simulink model "atrias_nmm_hardware"  (R2014b)
settings: Solver=FixedStepDiscrete  StartTime=0.0  StopTime=inf  FixedStep=sample_time  RelTol=1e-3
undefined symbols (not defined in the file or in its folder): A_lpf_dtau, B1_lpf_dtau, B2_lpf_dtau, boom_mount_angle, boom_pelvis_offset_angle, c, c_jointstop, contactThr, control_start_time, D12_T, d_y_boom_com_offset, d_y_boom_hip_offset, eref, fcut_contact, FmaxBFSH, FmaxGLU, FmaxHAM, FmaxHFL, FmaxRF, FmaxVAS, g, h_boom, HIP_MTR_MAX_CONT_TORQUE, initial_com_height, initial_dx, K, k_sea, kd_lateral, kp_lateral, l_boom_projected, L_distribution_switch, L_hip_trq_desired, L_knee_trq_desired, L_sea_ctrl_switch, l_seg, L_stim_gain, L_stim_switch, l_yaw_center_to_pelvis, lambdaHip, lambdaKnee, lateral_offset, lateral_target_angle_left, lateral_target_angle_right, lateral_transition_force, loptBFSH, loptGLU, loptHAM, loptHFL, loptRF, loptVAS, lslackBFSH, lslackGLU, lslackHAM, lslackHFL, lslackRF, lslackVAS, LStim_Constant, m_leg_motor, m_total_real, max_torque_lateral ... (+59)
libraries: simulink x5, simulink_extras x3, slrtlib x3
(part 1 of 4)
settings Model: BufferReuse=off  Creator=wmartin  LastModifiedBy=ryan
settings SolverCC: EnableConcurrentExecution=on
settings DataIOCC: MaxDataPoints=1000000000  SaveFormat=StructureWithTime
settings OptimizationCC: BlockReduction=off  OptimizeBlockIOStorage=off  BufferReuse=off  GlobalBufferReuse=off  ExpressionFolding=off  ExpressionDepthLimit=2147483647  LocalBlockOutputs=off  SimCompilerOptimization=On
settings DebuggingCC: UnderspecifiedInitializationDetection=Classic  MergeDetectMultiDrivingBlocksExec=none  StateNameClashWarn=warning
settings HardwareCC: ProdIntDivRoundTo=Zero  ProdEndianess=LittleEndian  ProdLongLongMode=on  ProdHWDeviceType=Generic->32-bit x86 compatible
settings ModelReferenceCC: UpdateModelReferenceTargets=IfOutOfDate  EnableParallelModelReferenceBuilds=on
settings RTWCC: SystemTargetFile=slrt.tlc  TemplateMakefile=slrt_default_tmf  Description=Simulink Real-Time  RTWVerbose=off  ProcessScript=slrt_make_rtw_hook  RTWCompilerOptimization=On
settings CodeAppCC: MaxIdLength=256
settings SimulinkRealTimeCC: GeneratePreprocessorConditionals=Disable all  EnableShiftOperators=on  RL32LogBufSizeModifier=100000000

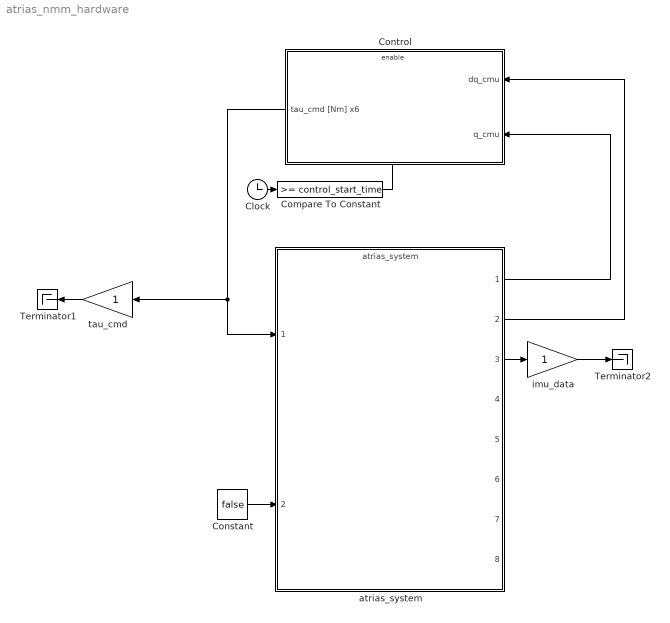
== system atrias_nmm_hardware ==
  Clock : Clock
  Compare To Constant : simulink/Logic and Bit Operations/Compare To Constant  relop=>=  const=control_start_time  OutDataTypeStr=boolean
  Constant : Constant  Value=false
  Control : Subsystem
  Terminator1 : Terminator
  Terminator2 : Terminator
  atrias_system : ModelReference  ModelNameDialog=atrias_system  SimulationMode=Normal  ModelReferenceVersion=1.2605  CopyOfModelName=atrias_system  DefaultDataLogging=on
  imu_data : Gain
  tau_cmd : Gain
  wires:
  Clock/1 -> Compare To Constant/1
  Compare To Constant/1 -> Control/Enable
  atrias_system/1 -> Control/2(q_cmu)
  atrias_system/2 -> Control/1(dq_cmu)
  Constant/1 -> atrias_system/2
  Control/1(tau_cmd [Nm] x6) -> tau_cmd/1, atrias_system/1
  imu_data/1 -> Terminator2/1
  atrias_system/3 -> imu_data/1
  tau_cmd/1 -> Terminator1/1

== system atrias_nmm_hardware/Control ==
  dq_cmu : Inport
  q_cmu : Inport  Port=2
  Enable : EnablePort  StatesWhenEnabling=reset
  Actuator Control : ModelReference  ModelNameDialog=actuator_control  SimulationMode=Normal  ModelReferenceVersion=1.66  CopyOfModelName=actuator_control  DefaultDataLogging=on
  Behavior Control : Subsystem
  tau_cmd [Nm] x6 : Outport  InitialOutput=[0 0 0 0 0 0]
  wires:
  q_cmu/1 -> Actuator Control/4, Behavior Control/2(q_cmu)
  dq_cmu/1 -> Actuator Control/5, Behavior Control/1(dq_cmu)
  Behavior Control/1(Motor Torque Command [Nm] x6) -> Actuator Control/1
  Actuator Control/1 -> tau_cmd [Nm] x6/1
  Behavior Control/2(SEA Torque Velocity Command [Nm] x4) -> Actuator Control/2
  Behavior Control/3(Force / Position Control [1/0] x4) -> Actuator Control/3

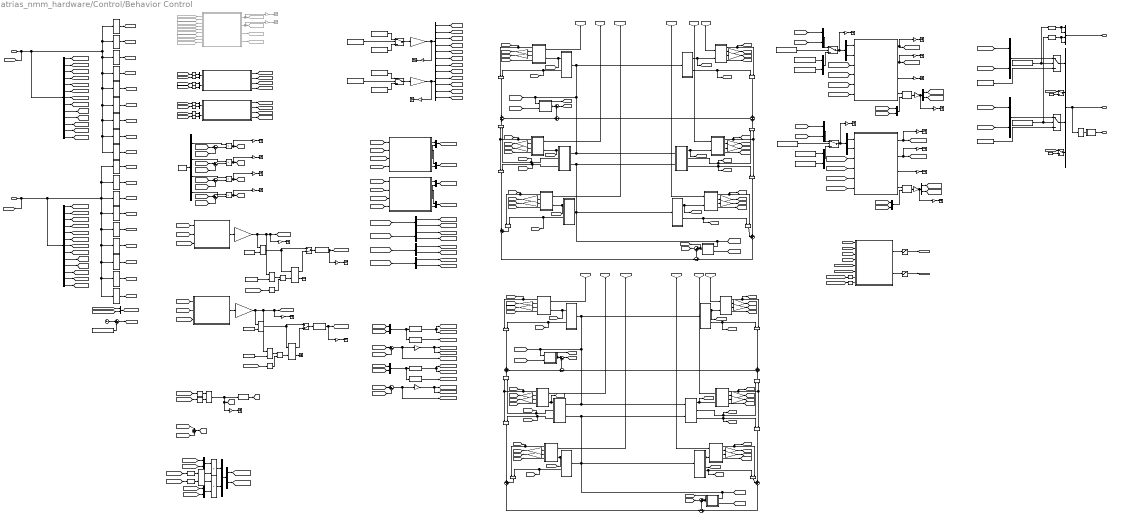
== system atrias_nmm_hardware/Control/Behavior Control ==
  note: Velocity Estimation
  note: Muscle Stimulation Input
  note: Leg/Spring Measurements
  note: Lateral Behavior
  note: Torque Commands
  note: Inputs
  note: q Order:
      |
      | backJointR
      | backGearR
      | frontJointR
      | frontGearR
      |
      | backJointL
      | backGearL
      | frontJointL
      | frontGearL
      |
      | latR
      | latL
      |
      | boomRoll
      | boomYaw
      | boomPitch
  note: Motor Order:
      |
      | backR
      | frontR
      | latR
      | backL
      | frontL
      | latL
  note: Muscle Geometry Input
  note: Atrias Knee/Splay Angles
  note: Estimate SEA Torque
  note: Estimate Leg Load and Contact
  note: Hip/Knee Torque Distribution
  note: Left Leg
  note: Neural Control Layer Interface
  note: Muscle Actuation Layer
  note: Body Mechanics Layer
      | Interface (Left Hip Joint)
  note: Body Mechanics Layer
      | Interface (Left Knee Joint)
  note: Right Leg
  note: Neural Control Layer Interface
  note: Body Mechanics Layer
      | Interface (Left Hip Joint)
  note: Body Mechanics Layer
      | Interface (Left Knee Joint)
  note: Estimate Flight/Escape
  note: Estimate GRFy
  note: Estimate Primary Leg Length/Angle
  dq_cmu : Inport
  q_cmu : Inport  Port=2
  Clock : Clock
  Constant : Constant  Value=0
  Constant1 : Constant  Value=0
  Constant10 : Constant  Value=releaseThr
  Constant11 : Constant  Value=contactThr
  Constant12 : Constant  Value=releaseThr
  Constant13 : Constant  Value=L_knee_trq_desired
  Constant14 : Constant  Value=R_knee_trq_desired
  Constant15 : Constant  Value=R_distribution_switch
  Constant16 : Constant  Value=L_distribution_switch
  Constant17 : Constant  Value=R_sea_ctrl_switch
  Constant18 : Constant  Value=L_sea_ctrl_switch
  Constant19 : Constant  Value=[0;0]
  Constant2 : Constant  Value=control_start_time
  Constant20 : Constant  Value=[0;0]
  Constant21 : Constant  Value=R_hip_trq_desired
  Constant22 : Constant  Value=L_hip_trq_desired
  Constant23 : Constant  Value=k_sea
  Constant3 : Constant  Value=LStim_Constant
  Constant4 : Constant  Value=RStim_Constant
  Constant5 : Constant  Value=[0;0;0;0;0;0]
  Constant6 : Constant  Value=[0;0;0;0;0;0]
  Constant7 : Constant  Value=R_stim_switch
  Constant8 : Constant  Value=L_stim_switch
  Constant9 : Constant  Value=contactThr
  Data Type Conversion : DataTypeConversion  OutDataTypeStr=double
  Data Type Conversion1 : DataTypeConversion  OutDataTypeStr=double
  Data Type Conversion{2..5} (4 alike) : DataTypeConversion  OutDataTypeStr=boolean
  Demux{,1,3,14..19} (9 alike) : Demux  Outputs=2
  Demux11 : Demux  Outputs=6
  Demux12 : Demux  Outputs=13
  Demux13 : Demux  Outputs=13
  Demux2 : Demux  Outputs=6
  Demux4 : Demux
  Detect Increase : simulink/Logic and Bit Operations/Detect Increase  vinit=0.0  InputProcessing=Inherited  OutDataTypeStr=boolean
  From116 : From  Commented=on  GotoTag=qBoomYaw
  From22 : From  Commented=on  GotoTag=GRFy
  From28 : From  Commented=on  GotoTag=dqBoomYaw
  From29 : From  Commented=on  GotoTag=qBoomRoll
  From45 : From  Commented=on  GotoTag=TorsoPitch
  From50 : From  Commented=on  GotoTag=PrimaryLegAngle
  From51 : From  Commented=on  GotoTag=PrimaryLegLength
  From52 : From  Commented=on  GotoTag=dqBoomRoll
  From81 : From  Commented=on  GotoTag=escape
  GLU Link : Subsystem
  GLU Link1 : Subsystem
  Gain : Gain
  Gain1 : Gain  Gain=R_stim_gain
  Gain2 : Gain  Gain=-1
  Gain3 : Gain  Gain=L_stim_gain
  Gain4 : Gain
  Gain5 : Gain  Gain=-1
  Goto26 : Goto  Commented=on  GotoTag=dx_avg
  Goto48 : Goto  Commented=on  GotoTag=dy_avg
  Goto49 : Goto  Commented=on  GotoTag=tApex
  Goto50 : Goto  Commented=on  GotoTag=systemEnergy
  HAM Link : Subsystem
  HAM Link1 : Subsystem
  HFL Link : Subsystem
  HFL Link1 : Subsystem
  L BFSH : Subsystem
  L BFSH Link : Subsystem
  L BFSH Link1 : Subsystem
  L GLU : Subsystem
  L Geometry : Subsystem
  L HAM : Subsystem
  L HFL : Subsystem
  L HFL Muscle Spindles{,1,4..5} (4 alike) : Gain  Gain=1/loptHFL
  L HFL Muscle Spindles{2..3,6..7} (4 alike) : Gain  Gain=1/loptGLU
  L Hip Joint Limits : Subsystem
  L Hip Joint Limits1 : Subsystem
  L Knee Joint Limits : Subsystem
  L Knee Joint Limits1 : Subsystem
  L Leg Calculator : Subsystem
  L Leg Load : Subsystem
  L RF : Subsystem
  L RF Muscle Spindles{,1..3} (4 alike) : Gain  Gain=1/loptRF
  L RF Muscle Spindles{4..7} (4 alike) : Gain  Gain=1/loptVAS
  L Torque : Subsystem
  L VAS : Subsystem
  LLoad : Gain
  L_Contact : Gain
  L_distribution_constraint_flag : Gain
  L_sea_B_des : Gain
  L_sea_B_meas : Gain
  L_sea_F_des : Gain
  L_sea_F_meas : Gain
  L_stim : Gain
  L_tau_virt_des : Gain
  L_tau_virt_meas : Gain
  Lateral Control : MATLAB Function  TreatAsAtomicUnit=on
  Left Lateral Torque Saturation : Saturate  UpperLimit=max_torque_lateral  LowerLimit=-max_torque_lateral
      settings: AttributesFormatString=Top: %<UpperLimit>\nBottom: %<LowerLimit>
  Logical Operator : Logic  Operator=NOT  AllPortsSameDT=off  OutDataTypeStr=boolean
  Logical Operator1 : Logic  AllPortsSameDT=off  OutDataTypeStr=boolean
  Logical Operator2 : Logic  AllPortsSameDT=off  OutDataTypeStr=boolean
  Logical Operator3 : Logic  Operator=NOT  AllPortsSameDT=off  OutDataTypeStr=boolean
  Logical Operator4 : Logic  AllPortsSameDT=off  OutDataTypeStr=boolean
  Manual Switch : ManualSwitch
  Manual Switch1 : ManualSwitch
  Manual Switch2 : ManualSwitch  CurrentSetting=0
  Manual Switch3 : ManualSwitch  CurrentSetting=0
  Matrix Multiply : Product  Multiplication=Matrix(*)
  Matrix Multiply1 : Product  Multiplication=Matrix(*)
  Memory : Memory
  Memory1 : Memory
  Mux : Mux
  Mux{1..2,4..13,17..18,20..27} (22 alike) : Mux  Inputs=2
  Mux3 : Mux
  Product{,1..3,10..11} (6 alike) : Product
  Product{4..9,12,14..15,17..23} (16 alike) : Product  RndMeth=Zero
  R BFSH : Subsystem
  R GLU : Subsystem
  R Geometry : Subsystem
  R HAM : Subsystem
  R HAM Muscle Spindles{1,3,6,14} (4 alike) : Gain  Gain=1/loptHAM
  R HAM Muscle Spindles{2,4,12..13} (4 alike) : Gain  Gain=1/loptBFSH
  R HFL : Subsystem
  R Leg Calculator : Subsystem
  R Leg Load : Subsystem
  R RF : Subsystem
  R Torque : Subsystem
  R VAS : Subsystem
  RF Link : Subsystem
  RF Link1 : Subsystem
  RLoad : Gain
  R_Contact : Gain
  R_distribution_constraint_flag : Gain
  R_sea_B_des : Gain
  R_sea_B_meas : Gain
  R_sea_F_des : Gain
  R_sea_F_meas : Gain
  R_stim : Gain
  R_tau_virt_des : Gain
  R_tau_virt_meas : Gain
  Relational Operator : RelationalOperator  OutDataTypeStr=boolean
  Relational Operator1 : RelationalOperator  Operator=<=  OutDataTypeStr=boolean
  Relational Operator2 : RelationalOperator  OutDataTypeStr=boolean
  Relational Operator3 : RelationalOperator  Operator=<=  OutDataTypeStr=boolean
  Right Lateral Torque Saturation : Saturate  UpperLimit=max_torque_lateral  LowerLimit=-max_torque_lateral
      settings: AttributesFormatString=Top: %<UpperLimit>\nBottom: %<LowerLimit>
  S-R Flip-Flop : simulink_extras/Flip Flops/S-R Flip-Flop  initial_condition=0
  S-R Flip-Flop1 : simulink_extras/Flip Flops/S-R Flip-Flop  initial_condition=0
  S-R Flip-Flop2 : simulink_extras/Flip Flops/S-R Flip-Flop  initial_condition=0
  Selector{,3,14..17,24..27} (10 alike) : Selector  InputPortWidth=2  Indices=[1]
  Selector1 : Selector  InputPortWidth=13  Indices=[10]
  Selector10 : Selector  InputPortWidth=13  Indices=[7 8]
  Selector11 : Selector  InputPortWidth=13  Indices=[9]
  Selector12 : Selector  InputPortWidth=13  Indices=[1 2]
  Selector13 : Selector  InputPortWidth=13  Indices=[3 4]
  Selector18 : Selector  InputPortWidth=13  Indices=[13]
  Selector2 : Selector  InputPortWidth=13  Indices=[5 6]
  Selector20 : Selector  InputPortWidth=13  Indices=[13]
  Selector21 : Selector  InputPortWidth=13  Indices=[11]
  Selector22 : Selector  InputPortWidth=13  Indices=[12]
  Selector23 : Selector  InputPortWidth=13  Indices=[11]
  Selector28 : Selector  InputPortWidth=13  Indices=[12]
  Selector33 : Selector  InputPortWidth=6  Indices=[1 2 4 5]
  Selector4 : Selector  InputPortWidth=13  Indices=[7 8]
  Selector5 : Selector  InputPortWidth=13  Indices=[9]
  Selector6 : Selector  InputPortWidth=13  Indices=[1 2]
  Selector7 : Selector  InputPortWidth=13  Indices=[3 4]
  Selector8 : Selector  InputPortWidth=13  Indices=[10]
  Selector9 : Selector  InputPortWidth=13  Indices=[5 6]
  Sum{,2,4,6,9,15,20} (7 alike) : Sum  Inputs=|+-
  Sum{1,7,12,16,18,22} (6 alike) : Sum  Inputs=|++
  Sum10 : Sum  Inputs=+-
  Sum{3,8,11,19,23} (5 alike) : Sum
  Sum13 : Sum  Inputs=++|
  Sum14 : Sum  Inputs=+-
  Sum17 : Sum  Inputs=++|
  Sum21 : Sum  Inputs=-+
  Sum5 : Sum  Inputs=-+
  Switch : Switch  Criteria=u2 ~= 0
  Switch1 : Switch  Criteria=u2 ~= 0
  Switch{2..5} (4 alike) : Switch  Criteria=u2 > Threshold
  Terminator : Terminator  Commented=on
  Terminator{1..4,6..24} (23 alike) : Terminator
  Terminator5 : Terminator  Commented=on
  VAS Link : Subsystem
  VAS Link1 : Subsystem
  Velocity Estimation : Subsystem  Commented=on
  "[N] to [%bw]" : Gain  Gain=1/(m_total_real*g)
  dtau_des : Subsystem
  dx_avg : Gain  Commented=on
  dy_avg : Gain  Commented=on
  flight : Gain
  knee angle : Fcn  Expr=pi-(u(1)-u(2))
  knee angle1 : Fcn  Expr=pi-(u(1)-u(2))
  percent body weight : Gain  Gain=1/(m_total_real*g)
  splay angle : Fcn  Expr=(u(1)-u(2))
  splay angle1 : Fcn  Expr=(u(1)-u(2))
  Motor Torque Command [Nm] x6 : Outport  OutputWhenDisabled=reset  InitialOutput=[0 0 0 0 0 0]
  SEA Torque Velocity Command [Nm] x4 : Outport  Port=2  OutputWhenDisabled=reset  InitialOutput=[0 0 0 0 0 0]
  Force / Position Control [1/0] x4 : Outport  Port=3  OutputWhenDisabled=reset  InitialOutput=[0 0 0 0 0 0]
  tag scope: GRFy=global, LActBFSH=global, LActGLU=global, LActHAM=global, LActHFL=global, LActRF=global, LActVAS=global, LFmBFSH=global, LFmGLU=global, LFmHAM=global, LFmHFL=global, LFmRF=global, LFmVAS=global, LFootCnt=global, LHipStop=global, LKneeStop=global, LLLoad=global, LLceBFSH=global, LLceGLU=global, LLceHAM=global, LLceHFL=global, LLceRF=global, LLceVAS=global, LLmtuBFSH=global, LLmtuGLU=global, LLmtuHAM=global, LLmtuHFL=global, LLmtuRF=global, LLmtuVAS=global, LM12=global, LM12_achieved=global, LM23=global, LM23_achieved=global, LStimBFSH=global, LStimGLU=global, LStimHAM=global, LStimHFL=global, LStimRF=global, LStimVAS=global, LVceBFSH=global, LVceGLU=global, LVceHAM=global, LVceHFL=global, LVceRF=global, LVceVAS=global, Ldgear_shin=global, Ldgear_thigh=global, Ldphi12=global, Ldphi23=global, Ldphi_Lat=global, Ldphi_back_knee=global, Ldphi_front_knee=global, Ldphi_lower_splay=global, Ldphi_shin=global, Ldphi_thigh=global, Lgear_shin=global, Lgear_thigh=global, Lphi12=global, Lphi12dphi12=global, Lphi23=global, Lphi23dphi23=global, Lphi_Lat=global, Lphi_back_knee=global, Lphi_front_knee=global, Lphi_lower_splay=global, Lphi_shin=global, Lphi_thigh=global, LrBFSH=global, LrGLU=global, LrHAMh=global, LrHAMk=global, LrHFL=global, LrRFh=global, LrRFk=global, LrVAS=global, Lshin_ctrl_trq=global, LtauB=global, LtauF=global, Lthigh_ctrl_trq=global, RActBFSH=global, RActGLU=global, RActHAM=global, RActHFL=global, RActRF=global, RActVAS=global, RFmBFSH=global, RFmGLU=global, RFmHAM=global, RFmHFL=global, RFmRF=global, RFmVAS=global, RFootCnt=global, RHipStop=global, RKneeStop=global, RLLoad=global, RLceBFSH=global, RLceGLU=global, RLceHAM=global, RLceHFL=global, RLceRF=global, RLceVAS=global, RLmtuBFSH=global, RLmtuGLU=global, RLmtuHAM=global, RLmtuHFL=global, RLmtuRF=global, RLmtuVAS=global, RM12=global, RM12_achieved=global, RM23=global, RM23_achieved=global, RStimBFSH=global, RStimGLU=global, RStimHAM=global, RStimHFL=global, RStimRF=global, RStimVAS=global, RVceBFSH=global, RVceGLU=global, RVceHAM=global, RVceHFL=global, RVceRF=global, RVceVAS=global, Rdgear_shin=global, Rdgear_thigh=global, Rdphi12=global, Rdphi23=global, Rdphi_Lat=global, Rdphi_back_knee=global, Rdphi_front_knee=global, Rdphi_lower_splay=global, Rdphi_shin=global, Rdphi_thigh=global, Rgear_shin=global, Rgear_thigh=global, Rphi12=global, Rphi12dphi12=global, Rphi23=global, Rphi23dphi23=global, Rphi_Lat=global, Rphi_back_knee=global, Rphi_front_knee=global, Rphi_lower_splay=global, Rphi_shin=global, Rphi_thigh=global, RrBFSH=global, RrGLU=global, RrHAMh=global, RrHAMk=global, RrHFL=global, RrRFh=global, RrRFk=global, RrVAS=global, Rshin_ctrl_trq=global, RtauB=global, RtauF=global, Rthigh_ctrl_trq=global, droll=global, dtheta=global, dyaw=global, escape=global, flight=global, roll=global, theta=global, yaw=global
  wires:
  Switch1/1 -> Mux/3
  Mux18/1 -> Switch1/1
  Constant19/1 -> Switch/3
  Mux17/1 -> Switch/1
  [Lthigh_ctrl_trq] -> Mux18/2
  [Lshin_ctrl_trq] -> Mux18/1
  [Rshin_ctrl_trq] -> Mux17/1
  [Rthigh_ctrl_trq] -> Mux17/2
  Manual Switch/1 -> Mux/4
  Manual Switch1/1 -> Mux/2
  Switch/1 -> Mux/1
  Constant18/1 -> Switch1/2, Data Type Conversion3/1
  Constant17/1 -> Switch/2, Data Type Conversion2/1
  Mux3/1 -> Force / Position Control [1/0] x4/1
  Mux7/1 -> [TorsoPitch]
  [dqBoomPitch] -> Mux7/2
  [qBoomPitch] -> Mux7/1
  Velocity Estimation/4(system_energy [J]) -> Goto50/1
  dy_avg/1 -> Terminator5/1
  Velocity Estimation/3(t_apex [s]) -> Goto49/1
  Velocity Estimation/2(dy_avg [m/s]) -> Goto48/1, dy_avg/1
  dx_avg/1 -> Terminator/1
  Velocity Estimation/1(dx_avg [m/s]) -> Goto26/1, dx_avg/1
  L Leg Calculator/4(w [m]) -> [LLegW]
  R Leg Calculator/4(w [m]) -> [RLegW]
  Selector26/1 -> Mux4/1
  Selector27/1 -> Mux4/2
  Selector25/1 -> Mux5/2
  Selector24/1 -> Mux5/1
  L Leg Calculator/3(Leg Splay [rad rad/s]) -> [LLegSplay]
  L Leg Calculator/2(Leg Angle [rad rad/s]) -> [LLegAngle]
  L Leg Calculator/1("Leg Length [m m/s] ") -> [LLegLength]
  Mux4/1 -> L Leg Calculator/2(Back [rad rad/s])
  Mux5/1 -> L Leg Calculator/1(Front [rad rad/s])
  [dqFrontL] -> Selector25/1
  [qFrontL] -> Selector24/1
  [dqBackL] -> Selector27/1
  [qBackL] -> Selector26/1
  Selector23/1 -> [qBoomRoll]
  Selector21/1 -> [dqBoomRoll]
  Selector22/1 -> [dqBoomYaw]
  Selector20/1 -> [dqBoomPitch]
  Selector18/1 -> [qBoomPitch]
  Selector16/1 -> Mux1/1
  Selector17/1 -> Mux1/2
  Selector15/1 -> Mux2/2
  Selector14/1 -> Mux2/1
  [tauLatL] -> Manual Switch/1
  [tauLatR] -> Manual Switch1/1
  R Leg Calculator/3(Leg Splay [rad rad/s]) -> [RLegSplay]
  R Leg Calculator/2(Leg Angle [rad rad/s]) -> [RLegAngle]
  R Leg Calculator/1("Leg Length [m m/s] ") -> [RLegLength]
  Mux1/1 -> R Leg Calculator/2(Back [rad rad/s])
  Mux2/1 -> R Leg Calculator/1(Front [rad rad/s])
  [dqFrontR] -> Selector15/1
  [qFrontR] -> Selector14/1
  [dqBackR] -> Selector17/1
  [qBackR] -> Selector16/1
  Selector10/1 -> [dqFrontL]
  Selector9/1 -> [dqBackL]
  Selector13/1 -> [dqFrontR]
  Selector12/1 -> [dqBackR]
  Selector11/1 -> [dqLatR]
  Selector8/1 -> [dqLatL]
  Constant/1 -> Manual Switch/2
  Constant1/1 -> Manual Switch1/2
  Clock/1 -> Sum/1
  Constant2/1 -> Sum/2
  Selector5/1 -> [qLatR]
  Selector1/1 -> [qLatL]
  Selector6/1 -> [qBackR]
  Selector7/1 -> [qFrontR]
  Selector2/1 -> [qBackL]
  Selector4/1 -> [qFrontL]
  Sum/1 -> [controlClock]
  Lateral Control/1(tau_r) -> Right Lateral Torque Saturation/1
  Lateral Control/2(tau_l) -> Left Lateral Torque Saturation/1
  Right Lateral Torque Saturation/1 -> [tauLatR]
  Left Lateral Torque Saturation/1 -> [tauLatL]
  Selector33/1 -> dtau_des/1(x)
  dtau_des/1(dx/dt) -> SEA Torque Velocity Command [Nm] x4/1
  Mux/1 -> Selector33/1, Motor Torque Command [Nm] x6/1
  [dqLatR] -> Lateral Control/2(dqLateralR)
  [qLatR] -> Lateral Control/1(qLateralR)
  [dqLatL] -> Lateral Control/4(dqLateralL)
  [qLatL] -> Lateral Control/3(qLateralL)
  [RLegLength] -> Selector/1
  [LLegLength] -> Selector3/1
  [RLegMeasuredForce] -> Lateral Control/5(F_leg_R)
  [LLegMeasuredForce] -> Lateral Control/6(F_leg_L)
  Selector/1 -> Lateral Control/7(L_leg_R)
  Selector3/1 -> Lateral Control/8(L_leg_L)
  From29/1 -> Velocity Estimation/1(qRoll [rad])
  From52/1 -> Velocity Estimation/2(dqRoll [rad/s])
  From45/1 -> Velocity Estimation/3(Torso Pitch [rad rad/s])
  From116/1 -> Velocity Estimation/4(qYaw [rad])
  From28/1 -> Velocity Estimation/5(dqYaw [rad/s])
  From22/1 -> Velocity Estimation/7(GRFy [body weight])
  From81/1 -> Velocity Estimation/6(escape [1/0])
  From51/1 -> Velocity Estimation/8(Primary Leg Length [m m/s])
  From50/1 -> Velocity Estimation/9(Primary Leg Angle [rad rad/s])
  Selector28/1 -> [qBoomYaw]
  Constant3/1 -> Switch3/1
  Demux2/1 -> [LStimHFL]
  Demux2/2 -> [LStimGLU]
  Demux2/3 -> [LStimHAM]
  Demux2/4 -> [LStimRF]
  Demux2/5 -> [LStimVAS]
  Demux2/6 -> [LStimBFSH]
  Constant4/1 -> Switch2/1
  Demux11/1 -> [RStimHFL]
  Demux11/2 -> [RStimGLU]
  Demux11/3 -> [RStimHAM]
  Demux11/4 -> [RStimRF]
  Demux11/5 -> [RStimVAS]
  Demux11/6 -> [RStimBFSH]
  Constant5/1 -> Switch2/3
  Constant6/1 -> Switch3/3
  Constant7/1 -> Switch2/2
  Constant8/1 -> Switch3/2
  Demux12/1 -> [Rphi_shin]
  Demux12/2 -> [Rgear_shin]
  Demux12/3 -> [Rphi_thigh]
  Demux12/4 -> [Rgear_thigh]
  Demux12/5 -> [Lphi_shin]
  Demux12/6 -> [Lgear_shin]
  Demux12/7 -> [Lphi_thigh]
  Demux12/8 -> [Lgear_thigh]
  Demux12/9 -> [Rphi_Lat]
  Demux12/10 -> [Lphi_Lat]
  Demux12/11 -> [roll]
  Demux12/12 -> [yaw]
  Demux12/13 -> [theta]
  q_cmu/1 -> Demux12/1, Selector1/1, Selector23/1, Selector28/1, Selector18/1, Selector5/1, Selector4/1, Selector2/1, Selector7/1, Selector6/1, [qCMU]
  dq_cmu/1 -> Demux13/1, Selector10/1, Selector11/1, Selector8/1, Selector21/1, Selector22/1, Selector20/1, Selector9/1, Selector13/1, Selector12/1, [dqCMU]
  Demux13/13 -> [dtheta]
  Demux13/8 -> [Ldgear_thigh]
  Demux13/10 -> [Ldphi_Lat]
  Demux13/6 -> [Ldgear_shin]
  Demux13/9 -> [Rdphi_Lat]
  Demux13/11 -> [droll]
  Demux13/12 -> [dyaw]
  Demux13/4 -> [Rdgear_thigh]
  Demux13/5 -> [Ldphi_shin]
  Demux13/7 -> [Ldphi_thigh]
  Demux13/1 -> [Rdphi_shin]
  Demux13/3 -> [Rdphi_thigh]
  Demux13/2 -> [Rdgear_shin]
  [Lphi_front_knee] -> L Leg Load/3(phi_12 [rad])
  L Leg Load/1(Leg Load [N]) -> "[N] to [%bw]"/1
  [LtauF] -> L Leg Load/1(tau_F [Nm])
  [LtauB] -> L Leg Load/2(tau_B [Nm])
  [Lphi_front_knee] -> L Torque/5(phi12 [rad])
  [Lphi23dphi23] -> L Torque/4(v23dv23 [rad,rad/s])
  [Lphi_thigh] -> L Torque/6(phi23 [rad])
  [Lphi12dphi12] -> L Torque/3("v12dv12 [rad, rad/s]")
  Matrix Multiply/1 -> Gain/1
  L Torque/4(Jinv [2x2]) -> Matrix Multiply/1
  [Lgear_shin] -> Sum6/1
  Sum6/1 -> Product10/2
  [Lphi_shin] -> Sum6/2
  [Lgear_thigh] -> Sum2/1
  Sum2/1 -> Product11/2
  [Lphi_thigh] -> Sum2/2
  Mux20/1 -> splay angle/1, knee angle/1
  [Lphi_thigh] -> Mux20/2
  [Lphi_shin] -> Mux20/1
  knee angle/1 -> [Lphi_back_knee], [Lphi_front_knee]
  [Ldphi_thigh] -> Sum4/2
  [Ldphi_shin] -> Sum4/1
  Sum4/1 -> Gain2/1, [Ldphi_lower_splay]
  Gain2/1 -> [Ldphi_back_knee], [Ldphi_front_knee]
  splay angle/1 -> [Lphi_lower_splay]
  Relational Operator/1 -> S-R Flip-Flop/1, Manual Switch2/1
  Constant9/1 -> Relational Operator/2
  S-R Flip-Flop/1 -> Manual Switch2/2
  S-R Flip-Flop/2 -> Terminator1/1
  Logical Operator1/1 -> S-R Flip-Flop/2
  [RFootCnt] -> Memory/1
  Constant10/1 -> Relational Operator1/2
  Relational Operator1/1 -> Logical Operator1/1
  Memory/1 -> Logical Operator1/2
  Mux21/1 -> Matrix Multiply/2
  [LtauF] -> Mux21/1
  [LtauB] -> Mux21/2
  Demux14/2 -> [LM23_achieved]
  Demux14/1 -> [LM12_achieved]
  Data Type Conversion/1 -> L_Contact/1, [LFootCnt]
  Manual Switch2/1 -> Data Type Conversion/1
  [Ldphi_front_knee] -> L Geometry/3(dphi12 [rad])
  [Ldphi_thigh] -> L Geometry/4(dphi23 [rad])
  [Lphi_thigh] -> L Geometry/2(phi23 [rad])
  [Lphi_front_knee] -> L Geometry/1(phi12 [rad])
  L Geometry/3(dv12 [rad/s]) -> Mux23/2
  L Geometry/4(dv23 [rad/s]) -> Mux22/2
  Mux23/1 -> [Lphi12dphi12]
  Mux22/1 -> [Lphi23dphi23]
  L Geometry/1(v12 [rad]) -> Mux23/1
  L Geometry/2(v23 [rad]) -> Mux22/1
  [Lphi12dphi12] -> Demux15/1
  Demux15/1 -> [Lphi12]
  Demux15/2 -> [Ldphi12]
  [Lphi23dphi23] -> Demux16/1
  Demux16/1 -> [Lphi23]
  Demux16/2 -> [Ldphi23]
  [Rphi_front_knee] -> R Leg Load/3(phi_12 [rad])
  R Leg Load/1(Leg Load [N]) -> percent body weight/1
  [RtauF] -> R Leg Load/1(tau_F [Nm])
  [RtauB] -> R Leg Load/2(tau_B [Nm])
  Mux24/1 -> splay angle1/1, knee angle1/1
  [Rphi_thigh] -> Mux24/2
  [Rphi_shin] -> Mux24/1
  knee angle1/1 -> [Rphi_back_knee], [Rphi_front_knee]
  [Rdphi_thigh] -> Sum15/2
  [Rdphi_shin] -> Sum15/1
  Sum15/1 -> [Rdphi_lower_splay], Gain5/1
  Gain5/1 -> [Rdphi_back_knee], [Rdphi_front_knee]
  splay angle1/1 -> [Rphi_lower_splay]
  [Rgear_shin] -> Sum20/1
  Sum20/1 -> Product2/2
  [Rphi_shin] -> Sum20/2
  [Rgear_thigh] -> Sum9/1
  Sum9/1 -> Product3/2
  [Rphi_thigh] -> Sum9/2
  Relational Operator2/1 -> S-R Flip-Flop1/1, Manual Switch3/1
  Constant11/1 -> Relational Operator2/2
  S-R Flip-Flop1/1 -> Manual Switch3/2
  S-R Flip-Flop1/2 -> Terminator3/1
  Logical Operator2/1 -> S-R Flip-Flop1/2
  [LFootCnt] -> Memory1/1
  Constant12/1 -> Relational Operator3/2
  Relational Operator3/1 -> Logical Operator2/1
  Memory1/1 -> Logical Operator2/2
  Manual Switch3/1 -> Data Type Conversion1/1
  [Rdphi_front_knee] -> R Geometry/3(dphi12 [rad])
  [Rdphi_thigh] -> R Geometry/4(dphi23 [rad])
  [Rphi_thigh] -> R Geometry/2(phi23 [rad])
  [Rphi_front_knee] -> R Geometry/1(phi12 [rad])
  R Geometry/1(v12 [rad]) -> Mux27/1
  R Geometry/3(dv12 [rad/s]) -> Mux27/2
  R Geometry/4(dv23 [rad/s]) -> Mux26/2
  Mux27/1 -> [Rphi12dphi12]
  Mux26/1 -> [Rphi23dphi23]
  R Geometry/2(v23 [rad]) -> Mux26/1
  [Rphi12dphi12] -> Demux18/1
  Demux18/1 -> [Rphi12]
  Demux18/2 -> [Rdphi12]
  [Rphi23dphi23] -> Demux19/1
  Demux19/1 -> [Rphi23]
  Demux19/2 -> [Rdphi23]
  [Rphi12dphi12] -> R Torque/3("v12dv12 [rad, rad/s]")
  [Rphi23dphi23] -> R Torque/4(v23dv23 [rad,rad/s])
  [Rphi_front_knee] -> R Torque/5(phi12 [rad])
  [Rphi_thigh] -> R Torque/6(phi23 [rad])
  Matrix Multiply1/1 -> Gain4/1
  R Torque/4(Jinv [2x2]) -> Matrix Multiply1/1
  Mux25/1 -> Matrix Multiply1/2
  [RtauF] -> Mux25/1
  [RtauB] -> Mux25/2
  Demux17/2 -> [RM23_achieved]
  Demux17/1 -> [RM12_achieved]
  Mux6/1 -> Switch4/1
  Constant15/1 -> Switch4/2
  [RM12] -> Mux6/1
  [RM23] -> Mux6/2
  Demux/1 -> R Torque/1(tau12_des [Nm])
  Demux/2 -> R Torque/2(tau23_des [Nm])
  Mux8/1 -> Switch5/1
  Constant16/1 -> Switch5/2
  [LM12] -> Mux8/1
  [LM23] -> Mux8/2
  Demux1/1 -> L Torque/1(tau12_des [Nm])
  Demux1/2 -> L Torque/2(tau23_des [Nm])
  Constant20/1 -> Switch1/3
  Mux9/1 -> Switch4/3
  Constant14/1 -> Mux9/1
  Constant21/1 -> Mux9/2
  Mux10/1 -> Switch5/3
  Constant13/1 -> Mux10/1
  Constant22/1 -> Mux10/2
  [Lphi12] -> L Knee Joint Limits/1(phi [rad]1), VAS Link/1(phi23 [rad]), RF Link/2(phi23 [rad]), HAM Link/2(phi23 [rad]), L BFSH Link/1(phi23 [rad])
  [LStimHAM] -> L HAM/1(STIM)
  L HAM/1(Fmtc) -> Product9/1, Product8/1, [LFmHAM]
  L HAM/2(Lce) -> R HAM Muscle Spindles1/1
  L HFL/1(Fmtc) -> Product7/2, [LFmHFL]
  L HFL/2(Lce) -> L HFL Muscle Spindles/1
  [LStimHFL] -> L HFL/1(STIM)
  L GLU/1(Fmtc) -> Product6/1, [LFmGLU]
  [LStimGLU] -> L GLU/1(STIM)
  Sum16/1 -> [LM23]
  [Ldphi12] -> L Knee Joint Limits/2(dphi [rad/s]1)
  VAS Link/1(lmtu [m]) -> [LLmtuVAS], L VAS/2(lmtc [m])
  HAM Link/1(lmtu [m]) -> [LLmtuHAM], L HAM/2(lmtc [m])
  HAM Link/2(lever34 [m]) -> Product8/2, [LrHAMh]
  HAM Link/3(lever23 [m]) -> Product9/2, [LrHAMk]
  Sum3/1 -> Sum14/1
  [Lphi23] -> L Hip Joint Limits/1(phi [rad]1), HFL Link/1(phi34 [rad]), GLU Link/1(phi34 [rad]), RF Link/1(phi34 [rad]), HAM Link/1(phi34 [rad])
  L VAS/4(A) -> [LActVAS]
  L VAS/1(Fmtc) -> Product4/2, [LFmVAS]
  Sum1/1 -> [LM12]
  L Knee Joint Limits/1(M_stop [Nm]1) -> Sum1/1, [LKneeStop]
  Sum5/1 -> Sum1/2
  VAS Link/2(lever [m]) -> [LrVAS], Product4/1
  Sum22/1 -> Sum5/1
  L HAM/4(A) -> [LActHAM]
  Product8/1 -> Sum3/2
  Product6/1 -> Sum3/1
  GLU Link/1(lmtu [m]) -> [LLmtuGLU], L GLU/2(lmtc [m])
  GLU Link/2(lever [m]) -> Product6/2, [LrGLU]
  L GLU/4(A) -> [LActGLU]
  [Ldphi23] -> L Hip Joint Limits/2(dphi [rad/s]1)
  L Hip Joint Limits/1(M_stop [Nm]1) -> [LHipStop], Sum16/1
  Sum14/1 -> Sum16/2
  HFL Link/1(lmtu [m]) -> [LLmtuHFL], L HFL/2(lmtc [m])
  L HFL/4(A) -> [LActHFL]
  HFL Link/2(lever [m]) -> Product7/1, [LrHFL]
  [LStimVAS] -> L VAS/1(STIM)
  L GLU/2(Lce) -> L HFL Muscle Spindles3/1
  L GLU/3(Vce) -> L HFL Muscle Spindles2/1
  L HAM/3(Vce) -> R HAM Muscle Spindles6/1
  L VAS/3(Vce) -> L RF Muscle Spindles6/1
  L VAS/2(Lce) -> L RF Muscle Spindles4/1
  L HFL/3(Vce) -> L HFL Muscle Spindles1/1
  L RF/4(A) -> [LActRF]
  L RF/3(Vce) -> L RF Muscle Spindles2/1
  L RF/2(Lce) -> L RF Muscle Spindles/1
  RF Link/1(lmtu [m]) -> [LLmtuRF], L RF/2(lmtc [m])
  RF Link/2(lever34 [m]) -> Product5/1, [LrRFh]
  RF Link/3(lever23 [m]) -> Product15/1, [LrRFk]
  [LStimRF] -> L RF/1(STIM)
  Product7/1 -> Sum11/1
  Product5/1 -> Sum11/2
  Product15/1 -> Sum17/2
  Sum17/1 -> Sum5/2
  Product4/1 -> Sum17/1
  [LStimBFSH] -> L BFSH/1(STIM)
  L BFSH Link/1(lmtu [m]) -> [LLmtuBFSH], L BFSH/2(lmtc [m])
  L BFSH Link/2(lever [m]) -> [LrBFSH], Product20/2
  L BFSH/4(A) -> [LActBFSH]
  L BFSH/2(Lce) -> R HAM Muscle Spindles4/1
  L BFSH/3(Vce) -> R HAM Muscle Spindles2/1
  Product20/1 -> Sum22/2
  Product9/1 -> Sum22/1
  L HFL Muscle Spindles1/1 -> [LVceHFL]
  L HFL Muscle Spindles2/1 -> [LVceGLU]
  L HFL Muscle Spindles3/1 -> [LLceGLU]
  L RF Muscle Spindles6/1 -> [LVceVAS]
  L RF/1(Fmtc) -> Product5/2, Product15/2, [LFmRF]
  L BFSH/1(Fmtc) -> Product20/1, [LFmBFSH]
  L HFL Muscle Spindles/1 -> [LLceHFL]
  R HAM Muscle Spindles1/1 -> [LLceHAM]
  R HAM Muscle Spindles6/1 -> [LVceHAM]
  L RF Muscle Spindles/1 -> [LLceRF]
  L RF Muscle Spindles2/1 -> [LVceRF]
  R HAM Muscle Spindles4/1 -> [LLceBFSH]
  R HAM Muscle Spindles2/1 -> [LVceBFSH]
  L RF Muscle Spindles4/1 -> [LLceVAS]
  [Rphi12] -> L Knee Joint Limits1/1(phi [rad]1), VAS Link1/1(phi23 [rad]), HAM Link1/2(phi23 [rad]), RF Link1/2(phi23 [rad]), L BFSH Link1/1(phi23 [rad])
  [RStimHAM] -> R HAM/1(STIM)
  R HAM/1(Fmtc) -> Product23/1, Product22/1, [RFmHAM]
  R HAM/2(Lce) -> R HAM Muscle Spindles3/1
  R HFL/1(Fmtc) -> Product21/2, [RFmHFL]
  R HFL/2(Lce) -> L HFL Muscle Spindles4/1
  [RStimHFL] -> R HFL/1(STIM)
  R GLU/1(Fmtc) -> Product19/1, [RFmGLU]
  [RStimGLU] -> R GLU/1(STIM)
  Sum12/1 -> [RM23]
  [Rdphi12] -> L Knee Joint Limits1/2(dphi [rad/s]1)
  VAS Link1/1(lmtu [m]) -> [RLmtuVAS], R VAS/2(lmtc [m])
  HAM Link1/1(lmtu [m]) -> [RLmtuHAM], R HAM/2(lmtc [m])
  HAM Link1/2(lever34 [m]) -> Product22/2, [RrHAMh]
  HAM Link1/3(lever23 [m]) -> Product23/2, [RrHAMk]
  Sum19/1 -> Sum10/1
  [Rphi23] -> L Hip Joint Limits1/1(phi [rad]1), HFL Link1/1(phi34 [rad]), GLU Link1/1(phi34 [rad]), RF Link1/1(phi34 [rad]), HAM Link1/1(phi34 [rad])
  R VAS/4(A) -> [RActVAS]
  R VAS/1(Fmtc) -> Product17/2, [RFmVAS]
  Sum7/1 -> [RM12]
  L Knee Joint Limits1/1(M_stop [Nm]1) -> Sum7/1, [RKneeStop]
  Sum21/1 -> Sum7/2
  VAS Link1/2(lever [m]) -> [RrVAS], Product17/1
  Sum18/1 -> Sum21/1
  R HAM/4(A) -> [RActHAM]
  Product22/1 -> Sum19/2
  Product19/1 -> Sum19/1
  GLU Link1/1(lmtu [m]) -> [RLmtuGLU], R GLU/2(lmtc [m])
  GLU Link1/2(lever [m]) -> Product19/2, [RrGLU]
  R GLU/4(A) -> [RActGLU]
  [Rdphi23] -> L Hip Joint Limits1/2(dphi [rad/s]1)
  L Hip Joint Limits1/1(M_stop [Nm]1) -> [RHipStop], Sum12/1
  Sum10/1 -> Sum12/2
  HFL Link1/1(lmtu [m]) -> [RLmtuHFL], R HFL/2(lmtc [m])
  R HFL/4(A) -> [RActHFL]
  HFL Link1/2(lever [m]) -> Product21/1, [RrHFL]
  [RStimVAS] -> R VAS/1(STIM)
  R GLU/2(Lce) -> L HFL Muscle Spindles7/1
  R GLU/3(Vce) -> L HFL Muscle Spindles6/1
  R HAM/3(Vce) -> R HAM Muscle Spindles14/1
  R VAS/3(Vce) -> L RF Muscle Spindles7/1
  R VAS/2(Lce) -> L RF Muscle Spindles5/1
  R HFL/3(Vce) -> L HFL Muscle Spindles5/1
  R RF/4(A) -> [RActRF]
  R RF/3(Vce) -> L RF Muscle Spindles3/1
  R RF/2(Lce) -> L RF Muscle Spindles1/1
  RF Link1/1(lmtu [m]) -> [RLmtuRF], R RF/2(lmtc [m])
  RF Link1/2(lever34 [m]) -> Product18/1, [RrRFh]
  RF Link1/3(lever23 [m]) -> [RrRFk], Product12/1
  [RStimRF] -> R RF/1(STIM)
  Sum8/1 -> Sum10/2
  Product21/1 -> Sum8/1
  Product18/1 -> Sum8/2
  Product12/1 -> Sum13/2
  Sum13/1 -> Sum21/2
  Product17/1 -> Sum13/1
  [RStimBFSH] -> R BFSH/1(STIM)
  L BFSH Link1/1(lmtu [m]) -> [RLmtuBFSH], R BFSH/2(lmtc [m])
  L BFSH Link1/2(lever [m]) -> [RrBFSH], Product14/2
  R BFSH/4(A) -> [RActBFSH]
  R BFSH/2(Lce) -> R HAM Muscle Spindles13/1
  R BFSH/3(Vce) -> R HAM Muscle Spindles12/1
  Product14/1 -> Sum18/2
  Product23/1 -> Sum18/1
  L HFL Muscle Spindles5/1 -> [RVceHFL]
  L HFL Muscle Spindles6/1 -> [RVceGLU]
  L HFL Muscle Spindles7/1 -> [RLceGLU]
  L RF Muscle Spindles7/1 -> [RVceVAS]
  R RF/1(Fmtc) -> Product18/2, Product12/2, [RFmRF]
  R BFSH/1(Fmtc) -> Product14/1, [RFmBFSH]
  L HFL Muscle Spindles4/1 -> [RLceHFL]
  R HAM Muscle Spindles3/1 -> [RLceHAM]
  R HAM Muscle Spindles14/1 -> [RVceHAM]
  L RF Muscle Spindles1/1 -> [RLceRF]
  L RF Muscle Spindles3/1 -> [RVceRF]
  R HAM Muscle Spindles13/1 -> [RLceBFSH]
  R HAM Muscle Spindles12/1 -> [RVceBFSH]
  L RF Muscle Spindles5/1 -> [RLceVAS]
  Sum11/1 -> Sum14/2
  [RFootCnt] -> Logical Operator/1
  [LFootCnt] -> Logical Operator3/1
  Logical Operator/1 -> Logical Operator4/1
  Logical Operator3/1 -> Logical Operator4/2
  Detect Increase/1 -> [escape]
  [RLLoad] -> Sum23/1
  [LLLoad] -> Sum23/2
  Sum23/1 -> [GRFy]
  [RLegLength] -> Mux11/1
  [RLegAngle] -> Mux11/2
  [LLegLength] -> Mux12/1
  [LLegAngle] -> Mux12/2
  [RFootCnt] -> Data Type Conversion4/1
  [LFootCnt] -> Data Type Conversion5/1
  S-R Flip-Flop2/2 -> Product1/1
  S-R Flip-Flop2/1 -> Product/2
  Mux11/1 -> Product/1
  Mux12/1 -> Product1/2
  Product/1 -> Mux13/1
  Product1/1 -> Mux13/2
  Mux13/1 -> Demux3/1
  Demux3/1 -> [PrimaryLegLength]
  Demux3/2 -> [PrimaryLegAngle]
  Constant23/1 -> Demux4/1
  Demux4/1 -> Product2/1
  Demux4/2 -> Product3/1
  Demux4/3 -> Product10/1
  Demux4/4 -> Product11/1
  L_Contact/1 -> Terminator2/1
  Data Type Conversion1/1 -> R_Contact/1, [RFootCnt]
  R_Contact/1 -> Terminator4/1
  Logical Operator4/1 -> Detect Increase/1, [flight], flight/1
  flight/1 -> Terminator6/1
  percent body weight/1 -> Relational Operator3/1, RLoad/1, [RLLoad], Relational Operator2/1
  RLoad/1 -> Terminator7/1
  "[N] to [%bw]"/1 -> Relational Operator/1, Relational Operator1/1, LLoad/1, [LLLoad]
  LLoad/1 -> Terminator8/1
  Switch2/1 -> Gain1/1
  R_stim/1 -> Terminator9/1
  Switch3/1 -> Gain3/1
  L_stim/1 -> Terminator10/1
  Switch4/1 -> R_tau_virt_des/1, Demux/1
  R_tau_virt_des/1 -> Terminator11/1
  Switch5/1 -> L_tau_virt_des/1, Demux1/1
  L_tau_virt_des/1 -> Terminator12/1
  Product2/1 -> R_sea_B_meas/1, [RtauB]
  R_sea_B_meas/1 -> Terminator13/1
  Product3/1 -> R_sea_F_meas/1, [RtauF]
  R_sea_F_meas/1 -> Terminator14/1
  Product10/1 -> L_sea_B_meas/1, [LtauB]
  L_sea_B_meas/1 -> Terminator15/1
  Product11/1 -> L_sea_F_meas/1, [LtauF]
  L_sea_F_meas/1 -> Terminator16/1
  Gain4/1 -> R_tau_virt_meas/1, Demux17/1
  R_tau_virt_meas/1 -> Terminator17/1
  Gain/1 -> L_tau_virt_meas/1, Demux14/1
  L_tau_virt_meas/1 -> Terminator18/1
  L Torque/2(tau_B [Nm]) -> L_sea_B_des/1, [Lshin_ctrl_trq]
  L_sea_B_des/1 -> Terminator19/1
  L Torque/1(tau_F [Nm]) -> L_sea_F_des/1, [Lthigh_ctrl_trq]
  L_sea_F_des/1 -> Terminator20/1
  R Torque/2(tau_B [Nm]) -> R_sea_B_des/1, [Rshin_ctrl_trq]
  R_sea_B_des/1 -> Terminator21/1
  R Torque/1(tau_F [Nm]) -> [Rthigh_ctrl_trq], R_sea_F_des/1
  R_sea_F_des/1 -> Terminator22/1
  Gain1/1 -> R_stim/1, Demux11/1
  Gain3/1 -> L_stim/1, Demux2/1
  Data Type Conversion2/1 -> Mux3/1, Mux3/2
  Data Type Conversion3/1 -> Mux3/3, Mux3/4
  Data Type Conversion4/1 -> S-R Flip-Flop2/1
  Data Type Conversion5/1 -> S-R Flip-Flop2/2
  R Torque/3(constraint flag [0/1]) -> R_distribution_constraint_flag/1
  R_distribution_constraint_flag/1 -> Terminator23/1
  L Torque/3(constraint_flag [0/1]) -> L_distribution_constraint_flag/1
  L_distribution_constraint_flag/1 -> Terminator24/1

== system atrias_nmm_hardware/Control/Behavior Control/GLU Link ==
  note: GLUTEUS Attachment
  phi34 [rad] : Inport
  Constant : Constant  Value=lslackGLU+loptGLU
  Constant1 : Constant  Value=rGLU
  Constant2 : Constant  Value=phirefGLU
  Gain2 : Gain  Gain=rhoGLU
  Product : Product  RndMeth=Zero
  Sum2 : Sum  Inputs=|+-
  Sum5 : Sum  Inputs=|+-
  lmtu [m] : Outport
  lever [m] : Outport  Port=2
  wires:
  Constant/1 -> Sum5/1
  Sum5/1 -> lmtu [m]/1
  Product/1 -> Gain2/1
  phi34 [rad]/1 -> Sum2/1
  Constant2/1 -> Sum2/2
  Sum2/1 -> Product/1
  Constant1/1 -> Product/2, lever [m]/1
  Gain2/1 -> Sum5/2

== system atrias_nmm_hardware/Control/Behavior Control/GLU Link1 ==
  note: GLUTEUS Attachment
  phi34 [rad] : Inport
  Constant : Constant  Value=lslackGLU+loptGLU
  Constant1 : Constant  Value=rGLU
  Constant2 : Constant  Value=phirefGLU
  Gain2 : Gain  Gain=rhoGLU
  Product : Product  RndMeth=Zero
  Sum2 : Sum  Inputs=|+-
  Sum5 : Sum  Inputs=|+-
  lmtu [m] : Outport
  lever [m] : Outport  Port=2
  wires:
  Constant/1 -> Sum5/1
  Sum5/1 -> lmtu [m]/1
  Product/1 -> Gain2/1
  phi34 [rad]/1 -> Sum2/1
  Constant2/1 -> Sum2/2
  Sum2/1 -> Product/1
  Constant1/1 -> Product/2, lever [m]/1
  Gain2/1 -> Sum5/2

== system atrias_nmm_hardware/Control/Behavior Control/HAM Link ==
  note: HAM Attachment
  phi34 [rad] : Inport
  phi23 [rad] : Inport  Port=2
  Constant1 : Constant  Value=rHAMk
  Constant2 : Constant  Value=phirefHAMk
  Constant3 : Constant  Value=rHAMh
  Constant4 : Constant  Value=lslackHAM+loptHAM
  Constant5 : Constant  Value=phirefHAMh
  Gain2 : Gain  Gain=rhoHAMh
  Gain4 : Gain  Gain=rhoHAMk
  Product : Product  RndMeth=Zero
  Product1 : Product  RndMeth=Zero
  Sum1 : Sum  Inputs=|+-
  Sum4 : Sum  Inputs=|+-
  Sum5 : Sum  Inputs=-++
  lmtu [m] : Outport
  lever34 [m] : Outport  Port=2
  lever23 [m] : Outport  Port=3
  wires:
  Sum5/1 -> lmtu [m]/1
  Constant4/1 -> Sum5/2
  Gain4/1 -> Sum5/3
  Gain2/1 -> Sum5/1
  phi34 [rad]/1 -> Sum4/1
  Constant5/1 -> Sum4/2
  Sum4/1 -> Product/1
  Constant3/1 -> Product/2, lever34 [m]/1
  Product/1 -> Gain2/1
  phi23 [rad]/1 -> Sum1/1
  Constant2/1 -> Sum1/2
  Sum1/1 -> Product1/1
  Constant1/1 -> Product1/2, lever23 [m]/1
  Product1/1 -> Gain4/1

== system atrias_nmm_hardware/Control/Behavior Control/HAM Link1 ==
  note: HAM Attachment
  phi34 [rad] : Inport
  phi23 [rad] : Inport  Port=2
  Constant1 : Constant  Value=rHAMk
  Constant2 : Constant  Value=phirefHAMk
  Constant3 : Constant  Value=rHAMh
  Constant4 : Constant  Value=lslackHAM+loptHAM
  Constant5 : Constant  Value=phirefHAMh
  Gain2 : Gain  Gain=rhoHAMh
  Gain4 : Gain  Gain=rhoHAMk
  Product : Product  RndMeth=Zero
  Product1 : Product  RndMeth=Zero
  Sum1 : Sum  Inputs=|+-
  Sum4 : Sum  Inputs=|+-
  Sum5 : Sum  Inputs=-++
  lmtu [m] : Outport
  lever34 [m] : Outport  Port=2
  lever23 [m] : Outport  Port=3
  wires:
  Sum5/1 -> lmtu [m]/1
  Constant4/1 -> Sum5/2
  Gain4/1 -> Sum5/3
  Gain2/1 -> Sum5/1
  phi34 [rad]/1 -> Sum4/1
  Constant5/1 -> Sum4/2
  Sum4/1 -> Product/1
  Constant3/1 -> Product/2, lever34 [m]/1
  Product/1 -> Gain2/1
  phi23 [rad]/1 -> Sum1/1
  Constant2/1 -> Sum1/2
  Sum1/1 -> Product1/1
  Constant1/1 -> Product1/2, lever23 [m]/1
  Product1/1 -> Gain4/1

== system atrias_nmm_hardware/Control/Behavior Control/HFL Link ==
  note: HFL Attachment
  phi34 [rad] : Inport
  Constant : Constant  Value=lslackHFL+loptHFL
  Constant1 : Constant  Value=rHFL
  Constant2 : Constant  Value=phirefHFL
  Gain2 : Gain  Gain=rhoHFL
  Product : Product  RndMeth=Zero
  Sum2 : Sum  Inputs=|+-
  Sum5 : Sum  Inputs=|++
  lmtu [m] : Outport
  lever [m] : Outport  Port=2
  wires:
  Constant/1 -> Sum5/1
  Sum5/1 -> lmtu [m]/1
  Product/1 -> Gain2/1
  phi34 [rad]/1 -> Sum2/1
  Constant2/1 -> Sum2/2
  Sum2/1 -> Product/1
  Constant1/1 -> Product/2, lever [m]/1
  Gain2/1 -> Sum5/2

== system atrias_nmm_hardware/Control/Behavior Control/HFL Link1 ==
  note: HFL Attachment
  phi34 [rad] : Inport
  Constant : Constant  Value=lslackHFL+loptHFL
  Constant1 : Constant  Value=rHFL
  Constant2 : Constant  Value=phirefHFL
  Gain2 : Gain  Gain=rhoHFL
  Product : Product  RndMeth=Zero
  Sum2 : Sum  Inputs=|+-
  Sum5 : Sum  Inputs=|++
  lmtu [m] : Outport
  lever [m] : Outport  Port=2
  wires:
  Constant/1 -> Sum5/1
  Sum5/1 -> lmtu [m]/1
  Product/1 -> Gain2/1
  phi34 [rad]/1 -> Sum2/1
  Constant2/1 -> Sum2/2
  Sum2/1 -> Product/1
  Constant1/1 -> Product/2, lever [m]/1
  Gain2/1 -> Sum5/2

== system atrias_nmm_hardware/Control/Behavior Control/L BFSH ==
  note: BFSH Muscle-Tendon Dynamics
  note: Excitation Contraction Coupling
  STIM : Inport
  lmtc [m] : Inport  Port=2
  1 : Product  Inputs=**  SaturateOnIntegerOverflow=on  InputSameDT=on  OutDataTypeStr=Inherit: Same as first input
  1/lslack : Gain  Gain=1/lslackBFSH  SaturateOnIntegerOverflow=on  OutDataTypeStr=Inherit: Same as input  ParamDataTypeStr=Inherit: Same as input
  BE force-length relation : Subsystem
  CE force-length relation : Subsystem
  CE inverse force-velocity relation : Subsystem
  Constant : Constant  Value=lslackBFSH
  Discrete ECC Transfer Function : DiscreteTransferFcn  Numerator=[1 1]  Denominator=[(1+2*tau/sample_time) (1-2*tau/sample_time)]  InitialStates=preA  SampleTime=sample_time
  Discrete-Time Integrator : DiscreteIntegrator  InitialConditionSource=external  InitialConditionSetting=State (most efficient)  SampleTime=sample_time
  Fmax : Gain  Gain=FmaxBFSH  SaturateOnIntegerOverflow=on  OutDataTypeStr=Inherit: Same as input  ParamDataTypeStr=Inherit: Same as input
  Fv = Fse / (A*Fce) : Product  Inputs=*/  SaturateOnIntegerOverflow=on  InputSameDT=on  OutDataTypeStr=Inherit: Same as first input
  PE force-length relation : Subsystem
  SE force-length relation : Subsystem
  Saturation : Saturate  UpperLimit=1  LowerLimit=0.01
  Sum : Sum  Inputs=|+-  SaturateOnIntegerOverflow=on  InputSameDT=on  OutDataTypeStr=Inherit: Same as first input
  Sum2 : Sum  Inputs=|-+  SaturateOnIntegerOverflow=on  InputSameDT=on  OutDataTypeStr=Inherit: Same as first input
  Sum3 : Sum  SaturateOnIntegerOverflow=on  InputSameDT=on  OutDataTypeStr=Inherit: Same as first input
  Sum4 : Sum  SaturateOnIntegerOverflow=on  InputSameDT=on  OutDataTypeStr=Inherit: Same as first input
  lce/lopt : Gain  Gain=1/loptBFSH  SaturateOnIntegerOverflow=on  OutDataTypeStr=Inherit: Same as input  ParamDataTypeStr=Inherit: Same as input
  vmax*lopt : Gain  Gain=vmaxBFSH*loptBFSH  SaturateOnIntegerOverflow=on  OutDataTypeStr=Inherit: Same as input  ParamDataTypeStr=Inherit: Same as input
  Fmtc : Outport  InitialOutput=0
  Lce : Outport  Port=2  InitialOutput=0
  Vce : Outport  Port=3  InitialOutput=0
  A : Outport  Port=4  InitialOutput=0
  wires:
  Discrete-Time Integrator/1 -> Sum/2, lce/lopt/1, Lce/1  "lce"
  Sum/1 -> 1/lslack/1  "lse"
  lce/lopt/1 -> CE force-length relation/1(lce [lopt]), BE force-length relation/1(lce [lopt]), PE force-length relation/1(lce [lopt])
  Fv = Fse / (A*Fce)/1 -> CE inverse force-velocity relation/1(Fv[Fmax])  "fv"
  vmax*lopt/1 -> Discrete-Time Integrator/1, Vce/1  "vce"
  lmtc [m]/1 -> Sum2/2, Sum/1  "lmtc"
  Fmax/1 -> Fmtc/1  "Fmtc"
  1/lslack/1 -> SE force-length relation/1(lse [lslack])
  SE force-length relation/1(fse [Fmax]) -> Fmax/1, Sum4/1
  Sum2/1 -> Discrete-Time Integrator/2
  Constant/1 -> Sum2/1
  CE force-length relation/1(fce [Fmax]) -> 1/1
  Sum4/1 -> Fv = Fse / (A*Fce)/1
  PE force-length relation/1(fpe [Fmax]) -> Sum3/1
  1/1 -> Sum3/2
  BE force-length relation/1(fbe [Fmax]) -> Sum4/2
  Sum3/1 -> Fv = Fse / (A*Fce)/2
  CE inverse force-velocity relation/1(v[vmax]) -> vmax*lopt/1
  STIM/1 -> Discrete ECC Transfer Function/1
  Discrete ECC Transfer Function/1 -> Saturation/1
  Saturation/1 -> A/1, 1/2

== system atrias_nmm_hardware/Control/Behavior Control/L BFSH Link ==
  note: BFSH Attachment
  phi23 [rad] : Inport
  Constant : Constant  Value=lslackBFSH+loptBFSH
  Constant1 : Constant  Value=rBFSH
  Constant2 : Constant  Value=phirefBFSH
  Gain4 : Gain  Gain=rhoBFSH
  Product : Product  RndMeth=Zero
  Sum2 : Sum  Inputs=|+-
  Sum5 : Sum  Inputs=|++
  lmtu [m] : Outport
  lever [m] : Outport  Port=2
  wires:
  Constant/1 -> Sum5/1
  Sum5/1 -> lmtu [m]/1
  Gain4/1 -> Sum5/2
  Product/1 -> Gain4/1
  phi23 [rad]/1 -> Sum2/1
  Constant2/1 -> Sum2/2
  Sum2/1 -> Product/1
  Constant1/1 -> Product/2, lever [m]/1

== system atrias_nmm_hardware/Control/Behavior Control/L BFSH Link1 ==
  note: BFSH Attachment
  phi23 [rad] : Inport
  Constant : Constant  Value=lslackBFSH+loptBFSH
  Constant1 : Constant  Value=rBFSH
  Constant2 : Constant  Value=phirefBFSH
  Gain4 : Gain  Gain=rhoBFSH
  Product : Product  RndMeth=Zero
  Sum2 : Sum  Inputs=|+-
  Sum5 : Sum  Inputs=|++
  lmtu [m] : Outport
  lever [m] : Outport  Port=2
  wires:
  Constant/1 -> Sum5/1
  Sum5/1 -> lmtu [m]/1
  Gain4/1 -> Sum5/2
  Product/1 -> Gain4/1
  phi23 [rad]/1 -> Sum2/1
  Constant2/1 -> Sum2/2
  Sum2/1 -> Product/1
  Constant1/1 -> Product/2, lever [m]/1

== system atrias_nmm_hardware/Control/Behavior Control/L GLU ==
  note: SOLEUS Muscle-Tendon Dynamics
  note: Excitation Contraction Coupling
  STIM : Inport
  lmtc [m] : Inport  Port=2
  1 : Product  Inputs=**  SaturateOnIntegerOverflow=on  InputSameDT=on  OutDataTypeStr=Inherit: Same as first input
  1/lslack : Gain  Gain=1/lslackGLU  SaturateOnIntegerOverflow=on  OutDataTypeStr=Inherit: Same as input  ParamDataTypeStr=Inherit: Same as input
  BE force-length relation : Subsystem
  CE force-length relation : Subsystem
  CE inverse force-velocity relation : Subsystem
  Constant : Constant  Value=lslackGLU
  Discrete ECC Transfer Function : DiscreteTransferFcn  Numerator=[1 1]  Denominator=[(1+2*tau/sample_time) (1-2*tau/sample_time)]  InitialStates=preA  SampleTime=sample_time
  Discrete-Time Integrator : DiscreteIntegrator  InitialConditionSource=external  InitialConditionSetting=State (most efficient)  SampleTime=sample_time
  Fmax : Gain  Gain=FmaxGLU  SaturateOnIntegerOverflow=on  OutDataTypeStr=Inherit: Same as input  ParamDataTypeStr=Inherit: Same as input
  Fv = Fse / (A*Fce) : Product  Inputs=*/  SaturateOnIntegerOverflow=on  InputSameDT=on  OutDataTypeStr=Inherit: Same as first input
  PE force-length relation : Subsystem
  SE force-length relation : Subsystem
  Saturation : Saturate  UpperLimit=1  LowerLimit=0.01
  Sum : Sum  Inputs=|+-  SaturateOnIntegerOverflow=on  InputSameDT=on  OutDataTypeStr=Inherit: Same as first input
  Sum2 : Sum  Inputs=|-+  SaturateOnIntegerOverflow=on  InputSameDT=on  OutDataTypeStr=Inherit: Same as first input
  Sum3 : Sum  SaturateOnIntegerOverflow=on  InputSameDT=on  OutDataTypeStr=Inherit: Same as first input
  Sum4 : Sum  SaturateOnIntegerOverflow=on  InputSameDT=on  OutDataTypeStr=Inherit: Same as first input
  lce/lopt : Gain  Gain=1/loptGLU  SaturateOnIntegerOverflow=on  OutDataTypeStr=Inherit: Same as input  ParamDataTypeStr=Inherit: Same as input
  vmax*lopt : Gain  Gain=vmaxGLU*loptGLU  SaturateOnIntegerOverflow=on  OutDataTypeStr=Inherit: Same as input  ParamDataTypeStr=Inherit: Same as input
  Fmtc : Outport  InitialOutput=0
  Lce : Outport  Port=2  InitialOutput=0
  Vce : Outport  Port=3  InitialOutput=0
  A : Outport  Port=4  InitialOutput=0
  wires:
  Discrete-Time Integrator/1 -> Sum/2, lce/lopt/1, Lce/1  "lce"
  Sum/1 -> 1/lslack/1  "lse"
  lce/lopt/1 -> CE force-length relation/1(lce [lopt]), BE force-length relation/1(lce [lopt]), PE force-length relation/1(lce [lopt])
  Fv = Fse / (A*Fce)/1 -> CE inverse force-velocity relation/1(Fv[Fmax])  "fv"
  vmax*lopt/1 -> Discrete-Time Integrator/1, Vce/1  "vce"
  lmtc [m]/1 -> Sum2/2, Sum/1  "lmtc"
  Fmax/1 -> Fmtc/1  "Fmtc"
  1/lslack/1 -> SE force-length relation/1(lse [lslack])
  SE force-length relation/1(fse [Fmax]) -> Fmax/1, Sum4/1
  Sum2/1 -> Discrete-Time Integrator/2
  Constant/1 -> Sum2/1
  CE force-length relation/1(fce [Fmax]) -> 1/1
  Sum4/1 -> Fv = Fse / (A*Fce)/1
  PE force-length relation/1(fpe [Fmax]) -> Sum3/1
  1/1 -> Sum3/2
  BE force-length relation/1(fbe [Fmax]) -> Sum4/2
  Sum3/1 -> Fv = Fse / (A*Fce)/2
  CE inverse force-velocity relation/1(v[vmax]) -> vmax*lopt/1
  STIM/1 -> Discrete ECC Transfer Function/1
  Discrete ECC Transfer Function/1 -> Saturation/1
  Saturation/1 -> A/1, 1/2

== system atrias_nmm_hardware/Control/Behavior Control/L Geometry ==
  note: Saturation prevents straight leg singularity
  phi12 [rad] : Inport
  phi23 [rad] : Inport  Port=2
  dphi12 [rad] : Inport  Port=3
  dphi23 [rad] : Inport  Port=4
  Constant : Constant  Value=D12_T
  Constant1 : Constant  Value=l_seg
  Divide : Product  Inputs=*/*
  Divide1 : Product  Inputs=**/*/
  Gain : Gain  Gain=2
  Gain{1..3,5} (4 alike) : Gain  Gain=0.5
  Sum : Sum  Inputs=|++
  Sum1 : Sum  Inputs=+-|
  Sum2 : Sum  Inputs=|++
  Sum3 : Sum  Inputs=|-+
  Trigonometric Function : Trigonometry  Operator=asin  OutputSignalType=real
  Trigonometric Function1 : Trigonometry
  Trigonometric Function3 : Trigonometry
  "[-1,1]" : Saturate  UpperLimit=1  LowerLimit=-1
  "[0,179°]" : Saturate  UpperLimit=v12_max  LowerLimit=0
  "[0.01,1]" : Saturate  UpperLimit=1  LowerLimit=0.01
  v12 [rad] : Outport
  v23 [rad] : Outport  Port=2
  dv12 [rad/s] : Outport  Port=3
  dv23 [rad/s] : Outport  Port=4
  wires:
  Constant1/1 -> Divide/1, Divide1/4  "l"
  Constant/1 -> Divide/2, Divide1/5  "lv"
  Trigonometric Function1/1 -> Divide/3
  Gain1/1 -> Trigonometric Function1/1
  phi12 [rad]/1 -> Gain1/1, Sum1/2, Gain3/1
  Gain/1 -> "[0,179°]"/1
  phi23 [rad]/1 -> Sum/2
  Sum1/1 -> Gain2/1
  Gain2/1 -> Sum/1
  Sum/1 -> v23 [rad]/1
  Divide/1 -> "[0.01,1]"/1, "[-1,1]"/1
  Trigonometric Function3/1 -> Divide1/2
  Trigonometric Function/1 -> Gain/1
  Gain3/1 -> Trigonometric Function3/1
  dphi12 [rad]/1 -> Sum3/1, Divide1/1
  Divide1/1 -> Sum3/2, dv12 [rad/s]/1
  dphi23 [rad]/1 -> Sum2/1
  Sum3/1 -> Gain5/1
  Gain5/1 -> Sum2/2
  Sum2/1 -> dv23 [rad/s]/1
  "[0,179°]"/1 -> v12 [rad]/1, Sum1/1
  "[0.01,1]"/1 -> Divide1/3
  "[-1,1]"/1 -> Trigonometric Function/1
